simulink subsystem "detector_obstaculos"  (R2023b)
settings: Solver=VariableStepAuto  StartTime=0.0  StopTime=10.0  RelTol=1e-3
libraries: simulink x2
settings Model: Creator=juana  LastModifiedBy=juana

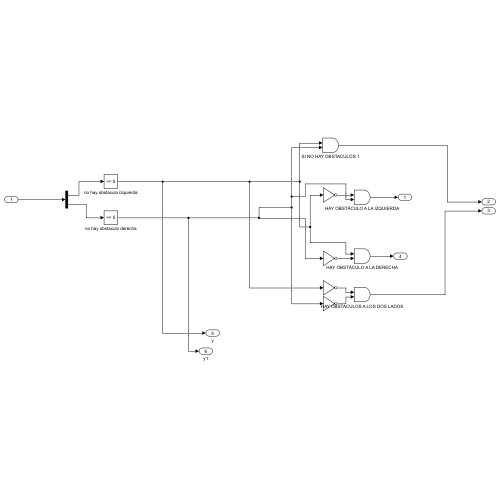
[thumbnail: Simulink's stored preview of the top-level diagram]
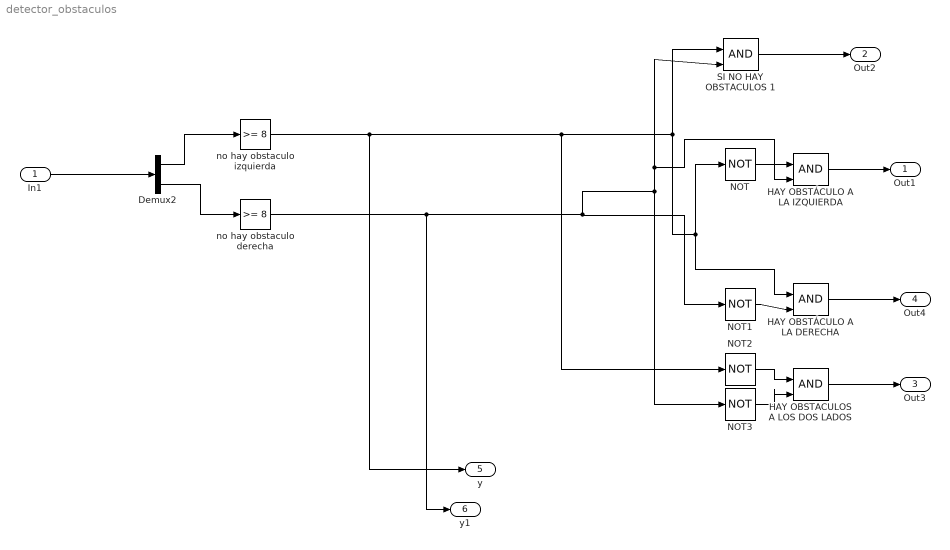
== system detector_obstaculos ==
  In1 : Inport
  Demux2 : Demux  Outputs=2
  HAY OBSTACULOS A LOS DOS LADOS : Logic  IconShape=distinctive  AllPortsSameDT=off  OutDataTypeStr=boolean
  HAY OBSTÁCULO A LA DERECHA : Logic  IconShape=distinctive  AllPortsSameDT=off  OutDataTypeStr=boolean
  HAY OBSTÁCULO A LA IZQUIERDA : Logic  IconShape=distinctive  AllPortsSameDT=off  OutDataTypeStr=boolean
  NOT{,1..3} (4 alike) : Logic  Operator=NOT  IconShape=distinctive  AllPortsSameDT=off  OutDataTypeStr=boolean
  SI NO HAY OBSTACULOS 1 : Logic  IconShape=distinctive  AllPortsSameDT=off  OutDataTypeStr=boolean
  no hay obstaculo derecha : simulink/Logic and Bit Operations/Compare To Constant  relop=>=  const=8  OutDataTypeStr=boolean
  no hay obstaculo izquierda : simulink/Logic and Bit Operations/Compare To Constant  relop=>=  const=8  OutDataTypeStr=boolean
  Out1 : Outport
  Out2 : Outport  Port=2
  Out3 : Outport  Port=3
  Out4 : Outport  Port=4
  y : Outport  Port=5
  y1 : Outport  Port=6
  wires:
  NOT1/1 -> HAY OBSTÁCULO A LA DERECHA/2
  no hay obstaculo izquierda/1 -> NOT2/1, NOT/1, HAY OBSTÁCULO A LA DERECHA/1, SI NO HAY OBSTACULOS 1/1, y/1
  no hay obstaculo derecha/1 -> NOT1/1, SI NO HAY OBSTACULOS 1/2, HAY OBSTÁCULO A LA IZQUIERDA/2, NOT3/1, y1/1
  NOT3/1 -> HAY OBSTACULOS A LOS DOS LADOS/2
  HAY OBSTÁCULO A LA DERECHA/1 -> Out4/1
  NOT2/1 -> HAY OBSTACULOS A LOS DOS LADOS/1
  HAY OBSTÁCULO A LA IZQUIERDA/1 -> Out1/1
  Demux2/1 -> no hay obstaculo izquierda/1
  NOT/1 -> HAY OBSTÁCULO A LA IZQUIERDA/1
  Demux2/2 -> no hay obstaculo derecha/1
  SI NO HAY OBSTACULOS 1/1 -> Out2/1
  HAY OBSTACULOS A LOS DOS LADOS/1 -> Out3/1
  In1/1 -> Demux2/1
